simulink model "fly_control"  (R2023a)
settings: Solver=VariableStepAuto  StartTime=0.0  StopTime=15.0  RelTol=1e-3
settings Model: DataDictionary=plane.sldd  Creator=Administrator  LastModifiedBy=Administrator
settings DataIOCC: ExternalInput="[cycle, joystickCmd,  rightAdverseYaw, leftAdverseYaw, OffPressed]"  LoadExternalInput=on  SaveFormat=Structure

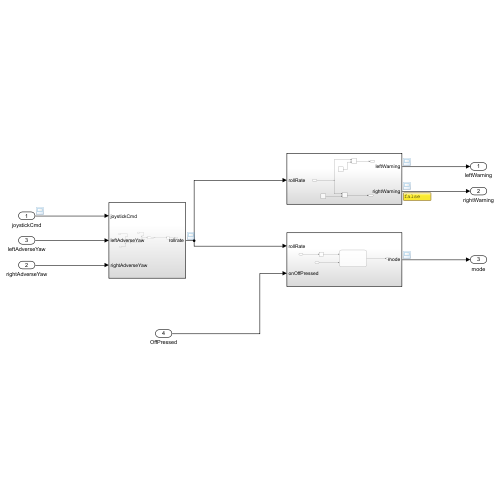
[thumbnail: Simulink's stored preview of the top-level diagram]
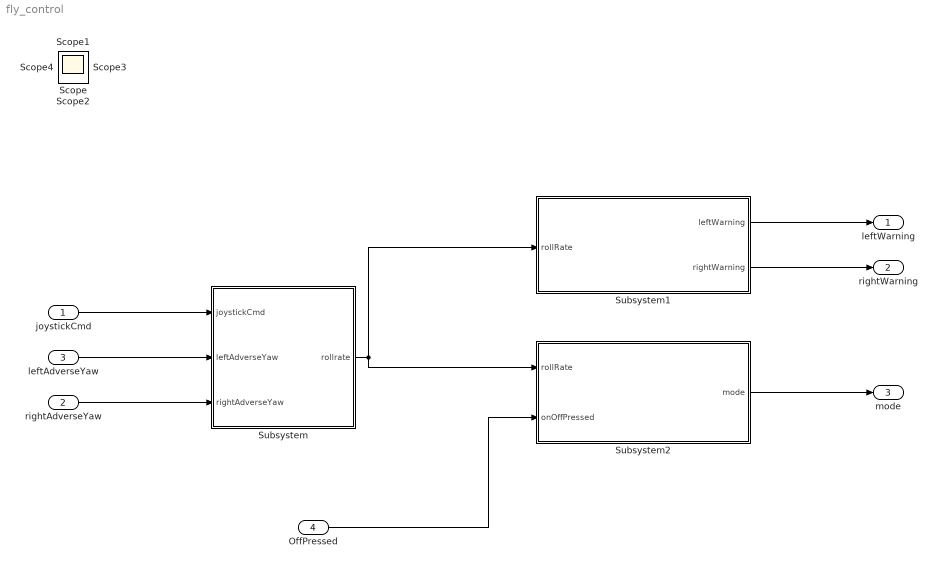
== system fly_control ==
  joystickCmd : Inport  OutDataTypeStr=double
  rightAdverseYaw : Inport  Port=2  OutDataTypeStr=double
  leftAdverseYaw : Inport  Port=3  OutDataTypeStr=double
  OffPressed : Inport  Port=4
  Subsystem : Subsystem
  Subsystem1 : Subsystem
  Subsystem2 : Subsystem
  leftWarning : Outport
  rightWarning : Outport  Port=2
  mode : Outport  Port=3
  Scope{,1..4} (5 alike) : Scope
  wires:
  leftAdverseYaw/1 -> Subsystem/2(leftAdverseYaw)
  rightAdverseYaw/1 -> Subsystem/3(rightAdverseYaw)
  joystickCmd/1 -> Subsystem/1(joystickCmd)
  Subsystem/1(rollrate) -> Subsystem2/1(rollRate), Subsystem1/1(rollRate)
  OffPressed/1 -> Subsystem2/2(onOffPressed)
  Subsystem1/1(leftWarning) -> leftWarning/1
  Subsystem1/2(rightWarning) -> rightWarning/1
  Subsystem2/1(mode) -> mode/1

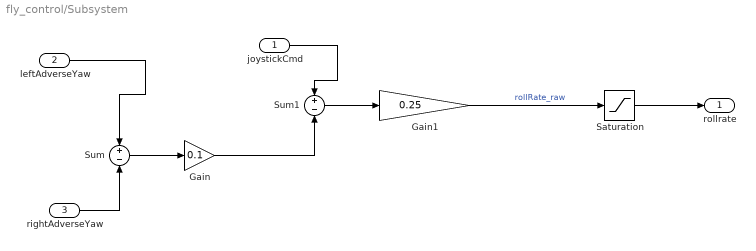
== system fly_control/Subsystem ==
  joystickCmd : Inport
  leftAdverseYaw : Inport  Port=2
  rightAdverseYaw : Inport  Port=3
  Gain : Gain  Gain=0.1
  Gain1 : Gain  Gain=0.25
  Saturation : Saturate  UpperLimit=25  LowerLimit=-25
  Sum : Sum  Inputs=+-
  Sum1 : Sum  Inputs=+-
  rollrate : Outport
  wires:
  Gain1/1 -> Saturation/1  "rollRate_raw"
  Gain/1 -> Sum1/2
  Sum1/1 -> Gain1/1
  Sum/1 -> Gain/1
  rightAdverseYaw/1 -> Sum/2
  joystickCmd/1 -> Sum1/1
  leftAdverseYaw/1 -> Sum/1
  Saturation/1 -> rollrate/1

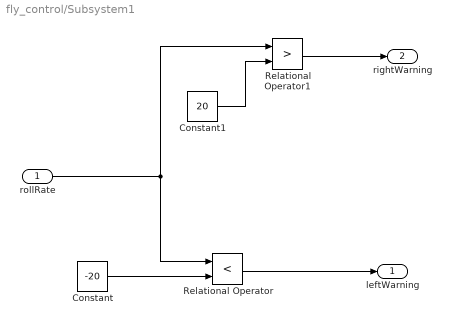
== system fly_control/Subsystem1 ==
  rollRate : Inport
  Constant : Constant  Value=-20
  Constant1 : Constant  Value=20
  Relational Operator : RelationalOperator  Operator=<  OutDataTypeStr=boolean  RndMeth=Simplest  InputSameDT=off
  Relational Operator1 : RelationalOperator  Operator=>  OutDataTypeStr=boolean  RndMeth=Simplest  InputSameDT=off
  leftWarning : Outport
  rightWarning : Outport  Port=2
  wires:
  Constant/1 -> Relational Operator/2
  rollRate/1 -> Relational Operator/1, Relational Operator1/1
  Relational Operator/1 -> leftWarning/1
  Constant1/1 -> Relational Operator1/2
  Relational Operator1/1 -> rightWarning/1

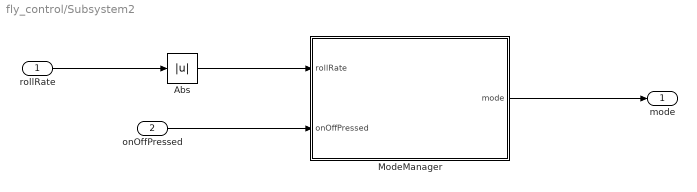
== system fly_control/Subsystem2 ==
  rollRate : Inport  OutDataTypeStr=double  PortDimensions=1
  onOffPressed : Inport  Port=2
  Abs : Abs  OutDataTypeStr=double  SaturateOnIntegerOverflow=off
  ModeManager : Stateflow chart  TreatAsAtomicUnit=on
  mode : Outport  OutDataTypeStr=Enum: modeEnum
  wires:
  onOffPressed/1 -> ModeManager/2(onOffPressed)
  ModeManager/1(mode) -> mode/1
  rollRate/1 -> Abs/1
  Abs/1 -> ModeManager/1(rollRate)

== stateflow chart fly_control/Subsystem2/ModeManager ==
  state NOMINAL
    entry:
    mode = modeEnum.NOMINAL;
  state OFF
    entry:
    mode = modeEnum.OFF;
  state FAILSOFT
    entry:
    mode = modeEnum.FAILSOFT;
  NOMINAL -> OFF [order 1] : [ onOffPressed ]
  OFF -> NOMINAL : [ onOffPressed && rollRate <= 20 ]
  NOMINAL -> FAILSOFT [order 2] : [ rollRate > kFailSoftRoll ]
  FAILSOFT -> NOMINAL : [ rollRate <= kFailSoftRoll ]
  (default) -> OFF
  data: rollRate input double size=1 [0..]; onOffPressed input size=1; mode output Enum: modeEnum; kFailSoftRoll constant double size=20
